simulink model "flex_att_dyn_mrp"  (R2020b)
settings: Solver=VariableStepAuto  StartTime=0.0  StopTime=10.0  RelTol=1e-3
undefined symbols (not defined in the file): bf, C, D, deta0, eta0, I, K, N, omega0, q0, Sf, t_final
settings Model: Creator=Amir  LastModifiedBy=Amir

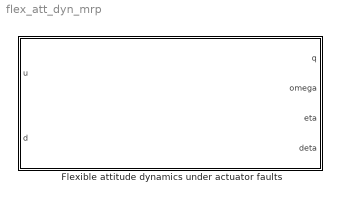
== system flex_att_dyn_mrp ==
  Flexible attitude dynamics under actuator faults : Subsystem  mask(Flexible Attitude Dynamics){I=I, I_copy=N, D=D, K=K, C=C, Sf=Sf, bf=bf, q0=q0, omega0=omega0, eta0=eta0, deta0=deta0}
      mask prompts: I "Inertia matrix (I):"; I_copy "Number of flexibility modes (N):"; D "Coupling matrix (D)"; K "Stiffness matrix (K):"; C "Damping matrix (C):"; Sf "Actuator fault scale factor (Sf):"; bf "Actuator fault bias (bf):"; q0 "Modified Rodrigues parameters (q0):"; omega0 "Angular velocity (omega0)"; eta0 "Modal coordinate vector (eta0)"; deta0 "Derivative of modal coordinate vector (deta0)"
      mask Help:
      | See the following paper for more details on the system:
      | 
      | C. Zhong, Z. Chen, Y. Guo, "Attitude control for  exible spacecraft with disturbance rejection", IEEE Transactions on Aerospace and Electronic Systems 53 (1) (2017) 101--110. doi: 10.1109/TAES.2017.2649259
      mask DialogControl DescGroupVar Prompt: Main
      mask DialogControl DescTextVar Prompt: Attitude dynamics of a flexible body (such as a spacecraft with elastic solar pannels), represented by modified Rodrigues parameters (MRPs). In the model, the effect of actuator faults, modeled by a scale factor matrix and a bias vector, are also taken into consideration.
      mask DialogControl ParameterGroupVar_copy Prompt: Initial Conditions
      mask Display:
      | image('$imagefile'); % Use "Edit Image" on toolstrip to change.
      | color('red'); port_label('output',1,'q (MRP)')
      | port_label('output',2,'omega (Angular velocity)')
      | port_label('output',3,'eta');port_label('output',4,'deta')
      | port_label('input',1,'u (Control input)')
      | port_label('input',2,'d (External disturbance torque)')

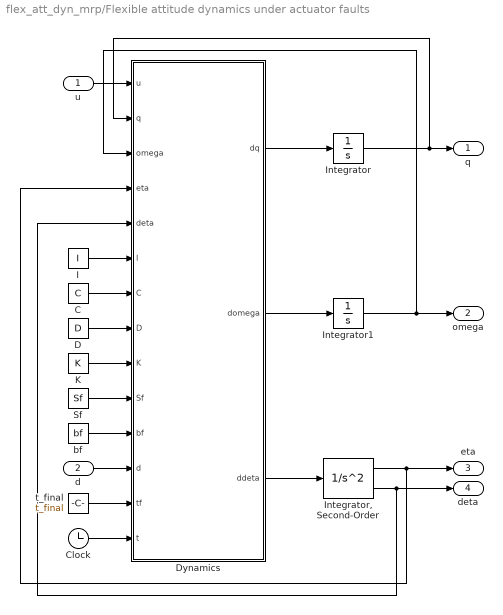
== system flex_att_dyn_mrp/Flexible attitude dynamics under actuator faults ==
  u : Inport
  d : Inport  Port=2
  C : Constant  Value=C
  Clock : Clock
  D : Constant  Value=D
  Dynamics : MATLAB Function  TreatAsAtomicUnit=on
  I : Constant  Value=I
  Integrator : Integrator  InitialCondition=q0
  "Integrator, Second-Order" : SecondOrderIntegrator  ICX=eta0  ICDXDT=deta0
  Integrator1 : Integrator  InitialCondition=omega0
  K : Constant  Value=K
  Sf : Constant  Value=Sf
  bf : Constant  Value=bf
  t_final : Constant  Value=t_final
  q : Outport
  omega : Outport  Port=2
  eta : Outport  Port=3
  deta : Outport  Port=4
  wires:
  u/1 -> Dynamics/1(u)
  Dynamics/1(dq) -> Integrator/1
  Dynamics/2(domega) -> Integrator1/1
  Integrator1/1 -> Dynamics/3(omega), omega/1
  Dynamics/3(ddeta) -> "Integrator, Second-Order"/1
  "Integrator, Second-Order"/1 -> Dynamics/4(eta), eta/1
  "Integrator, Second-Order"/2 -> deta/1, Dynamics/5(deta)
  Integrator/1 -> q/1, Dynamics/2(q)
  d/1 -> Dynamics/12(d)
  I/1 -> Dynamics/6(I)
  C/1 -> Dynamics/7(C)
  D/1 -> Dynamics/8(D)
  K/1 -> Dynamics/9(K)
  Sf/1 -> Dynamics/10(Sf)
  bf/1 -> Dynamics/11(bf)
  t_final/1 -> Dynamics/13(tf)
  Clock/1 -> Dynamics/14(t)

== matlab function flex_att_dyn_mrp/Flexible attitude dynamics under actuator faults/Dynamics ==
  data: u input size=[3 1]; q input size=[3 1]; dq output size=[3 1]; omega input size=[3 1]; eta input size=[N 1]; domega output size=[3 1]; ddeta output size=[N 1]; deta input size=[N 1]; I input size=[3 3]; C input size=[N N]; D input size=[N 3]; K input size=[N N]; Sf input size=[3 3]; bf input size=[3 1]; d input size=[3 1]; tf input; t input
function [dq,domega,ddeta] = fcn(u,q,omega,eta,deta,I,C,D,K,Sf,bf,d,tf,t)

% if t<tf/2
%     
%     bf=zeros(3,1);
%     
% end

qbracket=[0    -q(3)  q(2)
          q(3)  0    -q(1)
         -q(2)  q(1)  0];
     
omegabracket=[0        -omega(3)  omega(2)
              omega(3)  0        -omega(1)
             -omega(2)  omega(1)  0];

Theta=0.5*(0.5*(1-q'*q)*eye(3)+qbracket+q*q');

dq=Theta*omega;

domega=(inv(I-D'*D))*(D'*(C*deta+K*eta)-omegabracket*(I*omega+D'*deta)+d+bf+Sf*u);

ddeta=-D*domega-K*eta-C*deta;
